simulink model "qam_math1"  (R2018a)
settings: Solver=VariableStepAuto  StartTime=0.0  StopTime=10.0  RelTol=1e-3
settings Model: Creator=berke  LastModifiedBy=berke

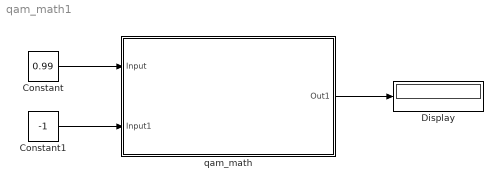
== system qam_math1 ==
  Constant : Constant  Value=0.99  OutDataTypeStr=fixdt(1,32,15)  SampleTime=0.1
  Constant1 : Constant  Value=-1  OutDataTypeStr=fixdt(1,2,0)  SampleTime=0.1
  Display : Display
  qam_math : Subsystem
  wires:
  qam_math/1(Out1) -> Display/1
  Constant/1 -> qam_math/1(Input)
  Constant1/1 -> qam_math/2(Input1)

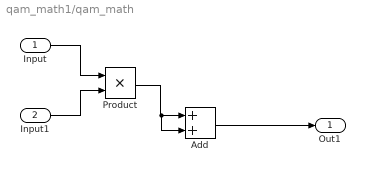
== system qam_math1/qam_math ==
  Input : Inport
  Input1 : Inport  Port=2
  Add : Sum
  Product : Product
  Out1 : Outport
  wires:
  Input1/1 -> Product/2
  Product/1 -> Add/2, Add/1
  Input/1 -> Product/1
  Add/1 -> Out1/1
